simulink model "SkywalkerX8_Control_Observable_Feedback"  (R2018a)
settings: Solver=FixedStepAuto  StartTime=0.0  StopTime=120  FixedStep=0.001  RelTol=1e-3
undefined symbols (not defined in the file): DiscIntNeverNeededParam, magnitude, sigbuilder_block, SkywalkerX8
libraries: simulink_extras x13, sensors x7, simulink x5, sharedTrackingLibrary x2, dspmtrx3 x1
(part 1 of 3)
settings Model: Creator=David  LastModifiedBy=David
settings SolverCC: AlgebraicLoopSolver=LineSearch

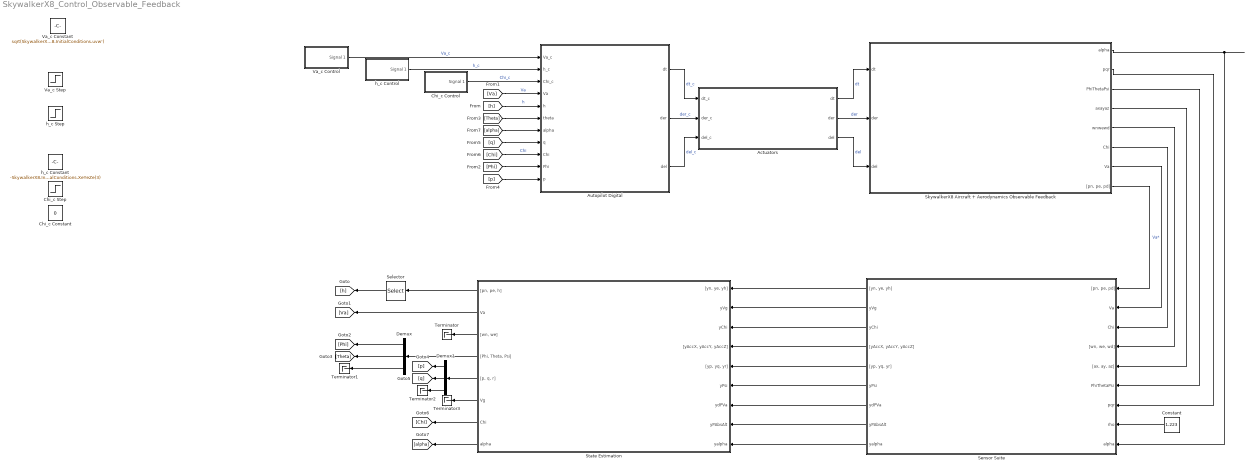
== system SkywalkerX8_Control_Observable_Feedback ==
  Actuators : Subsystem
      mask Display:
      | image('actuators.jpg', 'center')
      | 
      | color('white')
      | 
      | port_label('input', 1, 'd_{t_c} (Unitless)', 'texmode', 'on')
      | port_label('input', 2, 'd_{{er}_c} (rad)', 'texmode', 'on')
      | port_label('input', 3, 'd_{{el}_c} (rad)', 'texmode', 'on')
      | 
      | port_label('output', 1, 'd_t (Unitless)', 'texmode', 'on')
      | port_label('output', 2, 'd_{er} (rad)', 'texmode', 'on')
      | port_label('output', 3, 'd_{el} (rad)', 'texmode', 'on')
  Autopilot Digital : Subsystem
      mask Display:
      | image('autopilot.png', 'center')
      | 
      | port_label('output', 1, '\delta_t (Unitless)', 'texmode', 'on')
      | port_label('output', 2, '\delta_e_r (rad)', 'texmode', 'on')
      | port_label('output', 3, '\delta_e_l (rad)', 'texmode', 'on')
      | 
      | port_label('input', 1, 'V_{a_c} (m/s)', 'texmode', 'on')
      | port_label('input', 2, 'h_c (m)', 'texmode', 'on')
      | port_label('input', 3, '\chi_c (rad)', 'texmode', 'on')
      | port_label('input', 4, 'V_a (m/s)', 'texmode', 'on')
      | port_label('input', 5, 'Altitude (m)', 'texmode', 'on')
      | port_label('input', 6, '\theta (rad)', 'texmode', 'on')
      | port_label('input', 7, '\alpha (rad)', 'texmode', 'on')
      | port_label('input', 8, 'q (rad/s)', 'texmode', 'on')
      | port_label('input', 9, '\chi (rad)', 'texmode', 'on')
      | port_label('input', 10, '\phi (rad)', 'texmode', 'on')
      | port_label('input', 11, 'p (rad/s)', 'texmode', 'on')
  Chi_c Constant : Constant  Value=0
  Chi_c Control : Subsystem  Tag=STV Subsys  LoadFcn=sigbuilder_block('load');  StartFcn=sigbuilder_block('start');  StopFcn=sigbuilder_block('stop');  ClipboardFcn=sigbuilder_block('clipboard');  mask(Sigbuilder block){tuvar=[0:10]}
      mask help: Simulink:masks:SigbuilderBlock_MD
      mask init:
      | if ~strcmp(get_param(bdroot(gcbh),'SimulationStatus'),'stopped') tuvar = sigbuilder_block('maskInit'); end
      settings: CopyFcn=sigbuilder_block('copy');  DeleteFcn=sigbuilder_block('delete');  ModelCloseFcn=sigbuilder_block('modelClose');  PreSaveFcn=sigbuilder_block('preSave');  PauseFcn=sigbuilder_block('pause');  ContinueFcn=sigbuilder_block('continue');  NameChangeFcn=sigbuilder_block('namechange');  OpenFcn=sigbuilder_block('open',[437.6 199.2 550.4 400 ]);  CloseFcn=sigbuilder_block('close');
      mask Display: plot(0, 0, 100, 100,[2, 2, 32, 32, 2], [68, 8, 8, 68, 68],[32, 2], [38, 38], [32, 19, 2],[53, 60, 44], [32, 17, 17, 2],[16, 16, 31, 31]);txt = getActiveGroup(gcbh);text(2, 100, txt,'verticalAlignment', 'top');
  Chi_c Step : Step  After=deg2rad(90)  SampleTime=0
  Constant : Constant  Value=1.223
  Demux : Demux  Outputs=3
  Demux1 : Demux  Outputs=3
  Selector : Selector  InputPortWidth=3  IndexOptions=Index vector (dialog)  Indices=3  OutputSizes=1
  Sensor Suite : Subsystem
      mask Display:
      | image('telemetry.jpg')
      | 
      | color('cyan')
      | 
      | port_label('input', 1, '[p_N, p_E, p_D] (m)', 'texMode', 'On')
      | port_label('input', 2, 'V_a (m/s)', 'texMode', 'On')
      | port_label('input', 3, '\chi (rad)', 'texMode', 'On')
      | port_label('input', 4, '[w_N, w_E, w_D] (m/s)', 'texMode', 'On')
      | port_label('input', 5, '{\bfa_{inertial}} (m/s^2)', 'texMode', 'on')
      | port_label('input', 6, '[\phi, \theta, \psi] (rad)', 'texMode', 'on')
      | port_label('input', 7, '{\bf\omega_b} (rad/s)', 'texMode', 'on')
      | port_label('input', 8, '\rho (kg/m^3)', 'texMode', 'on')
      | port_label('input', 9, '\alpha (rad)', 'texMode', 'on')
      | 
      | port_label('output', 1, '[y_{GPS_N}, y_{GPS_E}, y_{GPS_h}] (m)', 'texMode', 'On')
      | port_label('output', 2, 'y_{GPS_{Vg}} (m/s)', 'texMode', 'On')
      | port_label('output', 3, 'y_{GPS_{\chi}} (rad)', 'texMode', 'On')
      | port_label('output', 4, '[y_{accel_x}, y_{accel_y}, y_{accel_z}] (m/s^2)', 'texMode', 'on')
      | port_label('output', 5, '[y_p, y_q, y_r] (rad/s)', 'texMode', 'on')
      | port_label('output', 6, 'y_{\psi} (rad)', 'texMode', 'on')
      | port_label('output', 7, 'y_{\DeltaP_{V_a}} (Pa)', 'texMode', 'on')
      | port_label('output', 8, 'y_{P_{abs}} (Pa)', 'texMode', 'on')
      | port_label('output', 9, 'y_\alpha (rad)', 'texMode', 'on')
  SkywalkerX8 Aircraft + Aerodynamics Observable Feedback : Subsystem
      mask Display:
      | image('x8SkySunset.png', 'center')
      | 
      | port_label('input', 1, '\delta_t (Unitless)', 'texmode', 'on')
      | port_label('input', 2, '\delta_e_r (rad)', 'texmode', 'on')
      | port_label('input', 3, '\delta_e_l (rad)', 'texmode', 'on')
      | 
      | port_label('output', 8, '[p_N, p_E, p_D] (m)', 'texMode', 'On')
      | port_label('output', 7, 'V_a (m/s)', 'texMode', 'On')
      | port_label('output', 6, '\chi (rad)', 'texMode', 'on')
      | port_label('output', 5, '[w_N, w_E, w_D] (m/s)', 'texMode', 'On')
      | port_label('output', 4, '{\bfa_{inertial}} (m/s^2)', 'texMode', 'on')
      | port_label('output', 3, '[\phi, \theta, \psi] (rad)', 'texMode', 'on')
      | port_label('output', 2, '{\bf\omega_b} (rad/s)', 'texMode', 'on')
      | port_label('output', 1, '\alpha (rad)', 'texMode', 'on')
  State Estimation : Subsystem
      mask Display:
      | image('state_estimate.jpg', 'center')
      | 
      | port_label('input', 1, '[y_{GPS_N}, y_{GPS_E}, y_{GPS_h}] (m)', 'texMode', 'On')
      | port_label('input', 2, 'y_{GPS_{Vg}} (m/s)', 'texMode', 'On')
      | port_label('input', 3, 'y_{GPS_{\chi}} (rad)', 'texMode', 'On')
      | port_label('input', 4, '[y_{accel_x}, y_{accel_y}, y_{accel_z}] (m/s^2)', 'texMode', 'on')
      | port_label('input', 5, '[y_p, y_q, y_r] (rad/s)', 'texMode', 'on')
      | port_label('input', 6, 'y_{\psi} (rad)', 'texMode', 'on')
      | port_label('input', 7, 'y_{\DeltaP_{V_a}} (Pa)', 'texMode', 'on')
      | port_label('input', 8, 'y_{P_{abs}} (Pa)', 'texMode', 'on')
      | port_label('input', 9, 'y_{\alpha} (rad)', 'texMode', 'on')
      | 
      | port_label('output', 1, '[p_N, p_E, h] (m)', 'texMode', 'On')
      | port_label('output', 2, 'V_a (m/s)', 'texMode', 'On')
      | port_label('output', 3, '[w_N, w_E] (m/s)', 'texMode', 'On')
      | port_label('output', 4, '[\phi, \theta, \psi] (rad)', 'texMode', 'on')
      | port_label('output', 5, '{\bf\omega_b} (rad/s)', 'texMode', 'on')
      | port_label('output', 6, 'V_g (m/s)', 'texMode', 'on')
      | port_label('output', 7, '\chi (rad)', 'texMode', 'on')
      | port_label('output', 8, '\alpha (rad)', 'texMode', 'on')
  Terminator{,1..3} (4 alike) : Terminator
  Va_c Constant : Constant  Value=sqrt(SkywalkerX8.InitialConditions.uvw*SkywalkerX8.InitialConditions.uvw')
  Va_c Control : Subsystem  Tag=STV Subsys  LoadFcn=sigbuilder_block('load');  StartFcn=sigbuilder_block('start');  StopFcn=sigbuilder_block('stop');  ClipboardFcn=sigbuilder_block('clipboard');  mask(Sigbuilder block){tuvar=[0:10]}
      mask help: Simulink:masks:SigbuilderBlock_MD
      mask init:
      | if ~strcmp(get_param(bdroot(gcbh),'SimulationStatus'),'stopped') tuvar = sigbuilder_block('maskInit'); end
      settings: CopyFcn=sigbuilder_block('copy');  DeleteFcn=sigbuilder_block('delete');  ModelCloseFcn=sigbuilder_block('modelClose');  PreSaveFcn=sigbuilder_block('preSave');  PauseFcn=sigbuilder_block('pause');  ContinueFcn=sigbuilder_block('continue');  NameChangeFcn=sigbuilder_block('namechange');  OpenFcn=sigbuilder_block('open',[437.6 199.2 550.4 400 ]);  CloseFcn=sigbuilder_block('close');
      mask Display: plot(0, 0, 100, 100,[2, 2, 32, 32, 2], [68, 8, 8, 68, 68],[32, 2], [38, 38], [32, 19, 2],[53, 60, 44], [32, 17, 17, 2],[16, 16, 31, 31]);txt = getActiveGroup(gcbh);text(2, 100, txt,'verticalAlignment', 'top');
  Va_c Step : Step  Before=sqrt(SkywalkerX8.InitialConditions.uvw*SkywalkerX8.InitialConditions.uvw')  After=sqrt(SkywalkerX8.InitialConditions.uvw*SkywalkerX8.InitialConditions.uvw')  SampleTime=0
  h_c Constant : Constant  Value=-SkywalkerX8.InitialConditions.XeYeZe(3)
  h_c Control : Subsystem  Tag=STV Subsys  LoadFcn=sigbuilder_block('load');  StartFcn=sigbuilder_block('start');  StopFcn=sigbuilder_block('stop');  ClipboardFcn=sigbuilder_block('clipboard');  mask(Sigbuilder block){tuvar=[0:10]}
      mask help: Simulink:masks:SigbuilderBlock_MD
      mask init:
      | if ~strcmp(get_param(bdroot(gcbh),'SimulationStatus'),'stopped') tuvar = sigbuilder_block('maskInit'); end
      settings: CopyFcn=sigbuilder_block('copy');  DeleteFcn=sigbuilder_block('delete');  ModelCloseFcn=sigbuilder_block('modelClose');  PreSaveFcn=sigbuilder_block('preSave');  PauseFcn=sigbuilder_block('pause');  ContinueFcn=sigbuilder_block('continue');  NameChangeFcn=sigbuilder_block('namechange');  OpenFcn=sigbuilder_block('open',[6 30 1428 771.75 ]);  CloseFcn=sigbuilder_block('close');
      mask Display: plot(0, 0, 100, 100,[2, 2, 32, 32, 2], [68, 8, 8, 68, 68],[32, 2], [38, 38], [32, 19, 2],[53, 60, 44], [32, 17, 17, 2],[16, 16, 31, 31]);txt = getActiveGroup(gcbh);text(2, 100, txt,'verticalAlignment', 'top');
  h_c Step : Step  Time=0.1  Before=-SkywalkerX8.InitialConditions.XeYeZe(3)  After=-2*SkywalkerX8.InitialConditions.XeYeZe(3)  SampleTime=0
  wires:
  Autopilot Digital/3(del) -> Actuators/3(del_c)  "del_c"
  Actuators/3(del) -> SkywalkerX8 Aircraft + Aerodynamics Observable Feedback/3(del)  "del"
  Actuators/2(der) -> SkywalkerX8 Aircraft + Aerodynamics Observable Feedback/2(der)  "der"
  Autopilot Digital/1(dt) -> Actuators/1(dt_c)  "dt_c"
  Chi_c Control/1(Signal 1) -> Autopilot Digital/3(Chi_c)  "Chi_c"
  Autopilot Digital/2(der) -> Actuators/2(der_c)  "der_c"
  h_c Control/1(Signal 1) -> Autopilot Digital/2(h_c)  "h_c"
  Actuators/1(dt) -> SkywalkerX8 Aircraft + Aerodynamics Observable Feedback/1(dt)  "dt"
  Va_c Control/1(Signal 1) -> Autopilot Digital/1(Va_c)  "Va_c"
  Sensor Suite/1("[yn, ye, yh]") -> State Estimation/1("[yn, ye, yh]")
  Sensor Suite/2(yVg) -> State Estimation/2(yVg)
  Sensor Suite/3(yChi) -> State Estimation/3(yChi)
  Sensor Suite/4("[yAccX, yAccY, yAccZ]") -> State Estimation/4("[yAccX, yAccY, yAccZ]")
  Sensor Suite/5("[yp, yq, yr]") -> State Estimation/5("[yp, yq, yr]")
  Sensor Suite/6(yPsi) -> State Estimation/6(yPsi)
  Sensor Suite/7(ydPVa) -> State Estimation/7(ydPVa)
  Sensor Suite/8(yPAbsAlt) -> State Estimation/8(yPAbsAlt)
  Sensor Suite/9(yalpha) -> State Estimation/9(yalpha)
  SkywalkerX8 Aircraft + Aerodynamics Observable Feedback/8("[pn, pe, pd]") -> Sensor Suite/1("[pn, pe, pd]")
  SkywalkerX8 Aircraft + Aerodynamics Observable Feedback/7(Va) -> Sensor Suite/2(Va)  "Va*"
  SkywalkerX8 Aircraft + Aerodynamics Observable Feedback/5(wnwewd) -> Sensor Suite/4("[wn, we, wd]")
  SkywalkerX8 Aircraft + Aerodynamics Observable Feedback/4(axayaz) -> Sensor Suite/5("[ax, ay, az]")
  SkywalkerX8 Aircraft + Aerodynamics Observable Feedback/3(PhiThetaPsi) -> Sensor Suite/6(PhiThetaPsi)
  SkywalkerX8 Aircraft + Aerodynamics Observable Feedback/2(pqr) -> Sensor Suite/7(pqr)
  SkywalkerX8 Aircraft + Aerodynamics Observable Feedback/1(alpha) -> Sensor Suite/9(alpha)
  Constant/1 -> Sensor Suite/8(rho)
  State Estimation/1("[pn, pe, h]") -> Selector/1
  Selector/1 -> [h]
  State Estimation/2(Va) -> [Va]
  State Estimation/3("[wn, we]") -> Terminator/1
  State Estimation/4("[Phi, Theta, Psi]") -> Demux/1
  Demux/1 -> [Phi]
  Demux/2 -> [Theta]
  Demux/3 -> Terminator1/1
  State Estimation/5("[p, q, r]") -> Demux1/1
  Demux1/1 -> [p]
  Demux1/2 -> [q]
  Demux1/3 -> Terminator2/1
  State Estimation/6(Vg) -> Terminator3/1
  State Estimation/7(Chi) -> [Chi]
  State Estimation/8(alpha) -> [alpha]
  [h] -> Autopilot Digital/5(h)  "h"
  [Va] -> Autopilot Digital/4(Va)  "Va"
  [Phi] -> Autopilot Digital/10(Phi)
  [Theta] -> Autopilot Digital/6(theta)
  [p] -> Autopilot Digital/11(p)
  [q] -> Autopilot Digital/8(q)
  [Chi] -> Autopilot Digital/9(Chi)  "Chi"
  [alpha] -> Autopilot Digital/7(alpha)
  SkywalkerX8 Aircraft + Aerodynamics Observable Feedback/6(Chi) -> Sensor Suite/3(Chi)

== system SkywalkerX8_Control_Observable_Feedback/Actuators ==
  dt_c : Inport
  der_c : Inport  Port=2
  del_c : Inport  Port=3
  Left Servo-Motor : Subsystem
      mask Display: image('servo.jpg', 'center')
  Motor Model : simulink_extras/Additional Linear/State-Space (with initial outputs)  A=SkywalkerX8.Actuators.Motor.SS.A  B=SkywalkerX8.Actuators.Motor.SS.B  C=SkywalkerX8.Actuators.Motor.SS.C  D=SkywalkerX8.Actuators.Motor.SS.D  U0=SkywalkerX8.InitialConditions.dt  Y0=SkywalkerX8.InitialConditions.dt  mask(State-Space with Initial Outputs){}
      settings: SourceProductName=Simulink  SourceProductBaseCode=SL
      mask Display: image('motor.jpg', 'center')
  Right Servo-Motor : Subsystem
      mask Display: image('servo.jpg', 'center')
  dt : Outport
  der : Outport  Port=2
  del : Outport  Port=3
  wires:
  del_c/1 -> Left Servo-Motor/1(del_c)
  Motor Model/1 -> dt/1
  Left Servo-Motor/1(del) -> del/1
  der_c/1 -> Right Servo-Motor/1(der_c)
  dt_c/1 -> Motor Model/1
  Right Servo-Motor/1(der) -> der/1

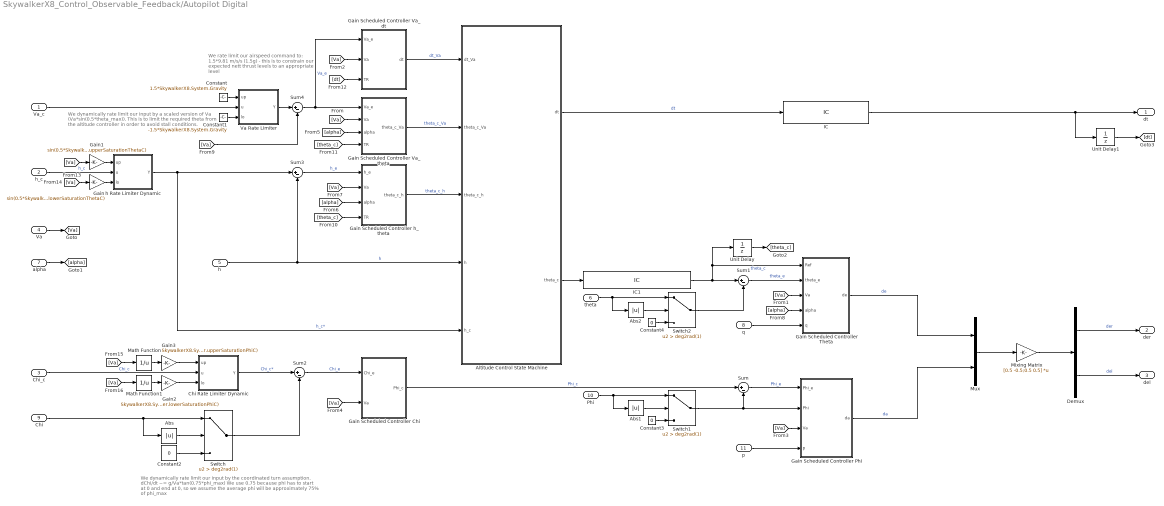
== system SkywalkerX8_Control_Observable_Feedback/Autopilot Digital ==
  note: We dynamically rate limit our input
      | by a scaled version of Va (Va*sin(0.5*theta_max)).
      |
      | This is to limit the required theta from the altitude controller
      | in order to avoid stall conditions.
  note: We dynamically rate limit our input
      | by the coordinated turn assumption.
      |
      | dChi/dt ~= g/Va*tan(0.75*phi_max)
      |
      | We use 0.75 because phi has to start at 0 and end at 0, so we assume
      | the average phi will be approximately 75% of phi_max
  note: We rate limit our airspeed command to:
      |
      | 1.5*9.81 m/s/s (1.5g) - this is to constrain our expected nett thrust levels to an appropriate level
  Va_c : Inport
  h_c : Inport  Port=2
  Chi_c : Inport  Port=3
  Va : Inport  Port=4
  h : Inport  Port=5
  theta : Inport  Port=6
  alpha : Inport  Port=7
  q : Inport  Port=8
  Chi : Inport  Port=9
  Phi : Inport  Port=10
  p : Inport  Port=11
  Abs : Abs
  Abs1 : Abs
  Abs2 : Abs
  Altitude Control State Machine : Stateflow chart  TreatAsAtomicUnit=on  mask{h_hold=SkywalkerX8.Control.Longitudinal.AltStateMachine.hHold, h_takeoff=SkywalkerX8.Control.Longitudinal.AltStateMachine.hTakeOff, theta_c_takeoff=SkywalkerX8.Control.Longitudinal.AltStateMachine.thetaTakeOff, hyst_frac=SkywalkerX8.Control.Longitudinal.AltStateMachine.HysteresisFraction, PreFlightBypass=SkywalkerX8.Control.Longitudinal.AltStateMachine.PreFlightBypass}
      mask prompts: h_hold "Altitude hold zone (+- band around the commanded altitude where theta will control altitude) (m)"; h_takeoff "Takeoff altitude (altitude after which we move away from constant pitch angle command) (m)"; theta_c_takeoff "Takeoff pitch angle (constant pitch angle at which to climb at at takeoff) (rad)"; hyst_frac "Hysteresis Fraction (Unitless)"; PreFlightBypass "Preflight Bypass (Unitless)"
  Chi Rate Limiter Dynamic : Subsystem  mask{initOutput=SkywalkerX8.InitialConditions.PhiThetaPsi(3)}
      mask prompts: initOutput "Initial output of dynamic rate limiter"
      mask DialogControl DescGroupVar Prompt: Rate Limiter Dynamic
      mask DialogControl DescTextVar Prompt: Limit rising and falling rates of the signals at the second input by using the first input (upper limit) and the third input (lower limit).
      mask Display:
      | image('rateLimit.png')
      | 
      | port_label('input', 1, 'up')
      | port_label('input', 2, 'u')
      | port_label('input', 3, 'lo')
      | 
      | port_label('output', 1, 'Y')
  Constant : Constant  Value=1.5*SkywalkerX8.System.Gravity
  Constant1 : Constant  Value=-1.5*SkywalkerX8.System.Gravity
  Constant2 : Constant  Value=0
  Constant3 : Constant  Value=0
  Constant4 : Constant  Value=0
  Demux : Demux  Outputs=2
  Gain : Gain  Gain=sin(0.5*SkywalkerX8.Control.Longitudinal.altController.lowerSaturationThetaC)
  Gain Scheduled Controller Chi : Subsystem
  Gain Scheduled Controller Phi : Subsystem
  Gain Scheduled Controller Theta : Subsystem
  Gain Scheduled Controller Va_dt : Subsystem
  Gain Scheduled Controller Va_theta : Subsystem
  Gain Scheduled Controller h_theta : Subsystem
  Gain1 : Gain  Gain=sin(0.5*SkywalkerX8.Control.Longitudinal.altController.upperSaturationThetaC)
  Gain2 : Gain  Gain=SkywalkerX8.System.Gravity*tan(0.75*SkywalkerX8.Control.Lateral.ChiController.lowerSaturationPhiC)
  Gain3 : Gain  Gain=SkywalkerX8.System.Gravity*tan(0.75*SkywalkerX8.Control.Lateral.ChiController.upperSaturationPhiC)
  IC : InitialCondition  Value=SkywalkerX8.InitialConditions.dt
  IC1 : InitialCondition  Value=SkywalkerX8.InitialConditions.PhiThetaPsi(2)
  Math Function : Math  Operator=reciprocal  SaturateOnIntegerOverflow=on
  Math Function1 : Math  Operator=reciprocal  SaturateOnIntegerOverflow=on
  Mixing Matrix : Gain  Gain=[0.5 -0.5;0.5 0.5]  Multiplication=Matrix(K*u)
  Mux : Mux  Inputs=2
  Sum{,1..4} (5 alike) : Sum  Inputs=|+-
  Switch : Switch  Criteria=u2 > Threshold  Threshold=deg2rad(1)
  Switch1 : Switch  Criteria=u2 > Threshold  Threshold=deg2rad(1)
  Switch2 : Switch  Criteria=u2 > Threshold  Threshold=deg2rad(1)
  Unit Delay : UnitDelay  InitialCondition=SkywalkerX8.InitialConditions.PhiThetaPsi(2)  SampleTime=SkywalkerX8.Control.Longitudinal.thetaController.Digital.SampleTime
  Unit Delay1 : UnitDelay  InitialCondition=SkywalkerX8.InitialConditions.dt  SampleTime=SkywalkerX8.Control.Longitudinal.VaDtController.Digital.SampleTime
  Va Rate Limiter : Subsystem  mask{initOutput=sqrt(SkywalkerX8.InitialConditions.uvw*SkywalkerX8.InitialConditions.uvw')}
      mask prompts: initOutput "Initial output of dynamic rate limiter"
      mask DialogControl DescGroupVar Prompt: Rate Limiter Dynamic
      mask DialogControl DescTextVar Prompt: Limit rising and falling rates of the signals at the second input by using the first input (upper limit) and the third input (lower limit).
      mask Display:
      | image('rateLimit.png')
      | 
      | port_label('input', 1, 'up')
      | port_label('input', 2, 'u')
      | port_label('input', 3, 'lo')
      | 
      | port_label('output', 1, 'Y')
  h Rate Limiter Dynamic : Subsystem  mask{initOutput=-SkywalkerX8.InitialConditions.XeYeZe(3)}
      mask prompts: initOutput "Initial output of dynamic rate limiter"
      mask DialogControl DescGroupVar Prompt: Rate Limiter Dynamic
      mask DialogControl DescTextVar Prompt: Limit rising and falling rates of the signals at the second input by using the first input (upper limit) and the third input (lower limit).
      mask Display:
      | image('rateLimit.png')
      | 
      | port_label('input', 1, 'up')
      | port_label('input', 2, 'u')
      | port_label('input', 3, 'lo')
      | 
      | port_label('output', 1, 'Y')
  dt : Outport
  der : Outport  Port=2
  del : Outport  Port=3
  wires:
  [Va] -> Sum4/2
  Sum4/1 -> Gain Scheduled Controller Va_theta/1(Va_e), Gain Scheduled Controller Va_dt/1(Va_e)  "Va_e"
  Demux/1 -> der/1  "der"
  Gain Scheduled Controller Chi/1(Phi_c) -> Sum/1  "Phi_c"
  h/1 -> Altitude Control State Machine/4(h), Sum3/2  "h"
  h Rate Limiter Dynamic/1(Y) -> Altitude Control State Machine/5(h_c), Sum3/1  "h_c*"
  Sum3/1 -> Gain Scheduled Controller h_theta/1(h_e)  "h_e"
  Sum2/1 -> Gain Scheduled Controller Chi/1(Chi_e)  "Chi_e"
  Switch1/1 -> Sum/2, Gain Scheduled Controller Phi/2(Phi)
  Sum/1 -> Gain Scheduled Controller Phi/1(Phi_e)  "Phi_e"
  Gain Scheduled Controller Phi/1(da) -> Mux/2  "da"
  [Va] -> Gain Scheduled Controller Phi/3(Va)
  [Va] -> Gain Scheduled Controller Theta/3(Va)
  Va_c/1 -> Va Rate Limiter/2(u)
  [alpha] -> Gain Scheduled Controller Va_theta/3(alpha)
  [Va] -> Gain Scheduled Controller Chi/2(Va)
  Sum1/1 -> Gain Scheduled Controller Theta/2(theta_e)  "theta_e"
  [Va] -> Gain Scheduled Controller Va_dt/2(Va)
  Demux/2 -> del/1  "del"
  alpha/1 -> [alpha]
  [Va] -> Gain Scheduled Controller Va_theta/2(Va)
  Chi/1 -> Abs/1, Switch/1
  Gain Scheduled Controller Theta/1(de) -> Mux/1  "de"
  p/1 -> Gain Scheduled Controller Phi/4(p)
  Va/1 -> [Va]
  Mux/1 -> Mixing Matrix/1
  Mixing Matrix/1 -> Demux/1
  [Va] -> Gain Scheduled Controller h_theta/2(Va)
  [alpha] -> Gain Scheduled Controller h_theta/3(alpha)
  Altitude Control State Machine/1(dt) -> IC/1  "dt"
  Gain Scheduled Controller Va_theta/1(theta_c_Va) -> Altitude Control State Machine/2(theta_c_Va)  "theta_c_Va"
  [theta_c] -> Gain Scheduled Controller Va_theta/4(TR)
  [dt] -> Gain Scheduled Controller Va_dt/3(TR)
  IC/1 -> Unit Delay1/1, dt/1
  [theta_c] -> Gain Scheduled Controller h_theta/4(TR)
  IC1/1 -> Unit Delay/1, Gain Scheduled Controller Theta/1(Ref), Sum1/1  "theta_c"
  [alpha] -> Gain Scheduled Controller Theta/4(alpha)
  q/1 -> Gain Scheduled Controller Theta/5(q)
  Gain Scheduled Controller h_theta/1(theta_c_h) -> Altitude Control State Machine/3(theta_c_h)  "theta_c_h"
  Altitude Control State Machine/2(theta_c) -> IC1/1
  Gain Scheduled Controller Va_dt/1(dt) -> Altitude Control State Machine/1(dt_Va)  "dt_Va"
  h_c/1 -> h Rate Limiter Dynamic/2(u)  "h_c"
  [Va] -> Gain1/1
  Gain/1 -> h Rate Limiter Dynamic/3(lo)
  [Va] -> Gain/1
  Gain1/1 -> h Rate Limiter Dynamic/1(up)
  [Va] -> Math Function1/1
  [Va] -> Math Function/1
  Gain2/1 -> Chi Rate Limiter Dynamic/3(lo)
  Gain3/1 -> Chi Rate Limiter Dynamic/1(up)
  Math Function/1 -> Gain3/1
  Math Function1/1 -> Gain2/1
  Va Rate Limiter/1(Y) -> Sum4/1
  Constant/1 -> Va Rate Limiter/1(up)
  Constant1/1 -> Va Rate Limiter/3(lo)
  Unit Delay/1 -> [theta_c]
  Unit Delay1/1 -> [dt]
  Abs/1 -> Switch/2
  Constant2/1 -> Switch/3
  Switch/1 -> Sum2/2
  Constant3/1 -> Switch1/3
  Abs1/1 -> Switch1/2
  Phi/1 -> Abs1/1, Switch1/1
  Constant4/1 -> Switch2/3
  Abs2/1 -> Switch2/2
  theta/1 -> Abs2/1, Switch2/1
  Switch2/1 -> Sum1/2
  Chi_c/1 -> Chi Rate Limiter Dynamic/2(u)  "Chi_c"
  Chi Rate Limiter Dynamic/1(Y) -> Sum2/1  "Chi_c*"

== system SkywalkerX8_Control_Observable_Feedback/Chi_c Control ==
  Demux : Demux  Tag=STV Demux  Outputs=1
  FromWs : FromWorkspace  Tag=STV FromWs  VariableName=tuvar  SampleTime=0
      SigBuilderData=|
      | common.afterFinalStr = 'Extrapolate'
      | common.sampleTime = 0
      | dataSet.timeRange = [0 120]
      | dataSet.name = 'Group 1'
      | sbobj.Groups.Name = 'Group 1'
      | sbobj.Groups.Signals.Name = 'Signal 1'
      | sbobj.Groups.Signals.XData = [0 10 10 35 35 55 55 90 90 120]
      | sbobj.Groups.Signals.YData = [0 0 1.5708 1.5708 0 0 1.5708 1.5708 0 0]
      | sbobj.Groups.TimeRange = [0 120]
  Signal 1 : Outport  Tag=STV Outport
  wires:
  Demux/1 -> Signal 1/1
  FromWs/1 -> Demux/1

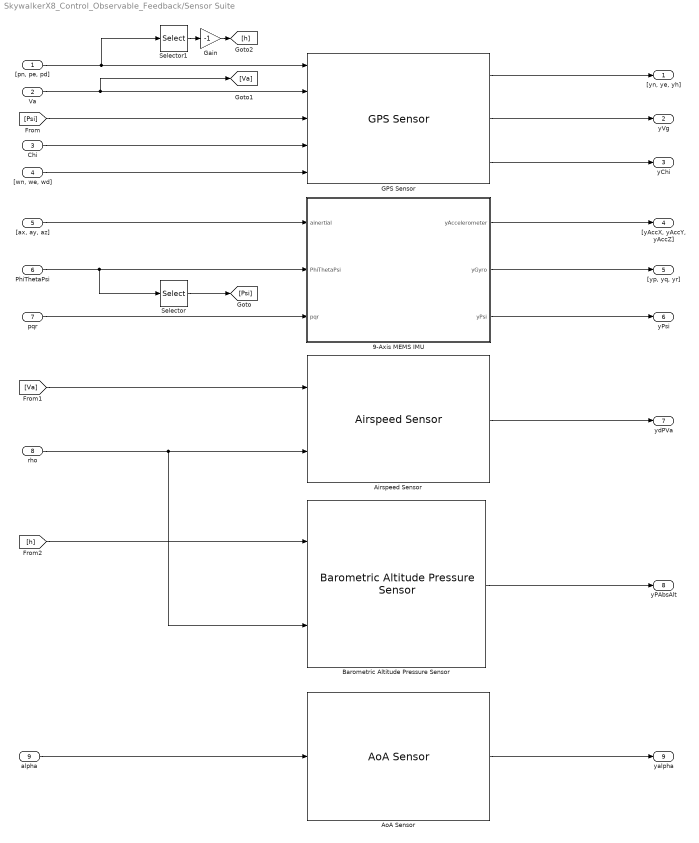
== system SkywalkerX8_Control_Observable_Feedback/Sensor Suite ==
  "[pn, pe, pd]" : Inport
  Va : Inport  Port=2
  Chi : Inport  Port=3
  "[wn, we, wd]" : Inport  Port=4
  "[ax, ay, az]" : Inport  Port=5
  PhiThetaPsi : Inport  Port=6
  pqr : Inport  Port=7
  rho : Inport  Port=8
  alpha : Inport  Port=9
  9-Axis MEMS IMU : Subsystem
      mask Display:
      | image('VNAV_IMU.jpg')
      | 
      | color('green')
      | 
      | port_label('input', 1, '{\bfa_{inertial}} (m/s^2)', 'texMode', 'on')
      | port_label('input', 2, '[\phi, \theta, \psi] (rad)', 'texMode', 'on')
      | port_label('input', 3, '{\bf\omega_b} (rad/s)', 'texMode', 'on')
      | 
      | port_label('output', 1, '[y_{accel_x}, y_{accel_y}, y_{accel_z}] (m/s^2)', 'texMode', 'on')
      | port_label('output', 2, '[y_p, y_q, y_r] (rad/s)', 'texMode', 'on')
      | port_label('output', 3, 'y_{\psi} (rad)', 'texMode', 'on')
  Airspeed Sensor : sensors/Airspeed Sensor  SampleTime=SkywalkerX8.Sensors.AirspeedPressure.SampleTime  diffPressureStdDev=SkywalkerX8.Sensors.AirspeedPressure.StdDev  diffPressureBandwidthHz=SkywalkerX8.Sensors.AirspeedPressure.BandwidthHz  diffPressureInit=SkywalkerX8.Sensors.AirspeedPressure.InitialCondition  diffPressureUpperSaturation=SkywalkerX8.Sensors.AirspeedPressure.UpperSat  diffPressureLowerSaturation=SkywalkerX8.Sensors.AirspeedPressure.LowerSat  diffPressureResolution=SkywalkerX8.Sensors.AirspeedPressure.Resolution
  AoA Sensor : sensors/AoA Sensor  SampleTime=SkywalkerX8.Sensors.AoA.SampleTime  alphaStdDev=SkywalkerX8.Sensors.AoA.StdDev  alphaBandwidthHz=SkywalkerX8.Sensors.AoA.BandwidthHz  alphaInit=SkywalkerX8.Sensors.AoA.InitialCondition  alphaUpperSaturation=SkywalkerX8.Sensors.AoA.UpperSat  alphaLowerSaturation=SkywalkerX8.Sensors.AoA.LowerSat  alphaResolution=SkywalkerX8.Sensors.AoA.Resolution
  Barometric Altitude Pressure Sensor : sensors/Barometric Altitude Pressure Sensor  g=SkywalkerX8.System.Gravity  SampleTime=SkywalkerX8.Sensors.AltitudePressure.SampleTime  absPressureStdDev=SkywalkerX8.Sensors.AltitudePressure.StdDev  absPressureBandwidthHz=SkywalkerX8.Sensors.AltitudePressure.BandwidthHz  absPressureInit=SkywalkerX8.Sensors.AltitudePressure.InitialCondition  absPressureUpperSaturation=SkywalkerX8.Sensors.AltitudePressure.UpperSat  absPressureLowerSaturation=SkywalkerX8.Sensors.AltitudePressure.LowerSat  absPressureResolution=SkywalkerX8.Sensors.AltitudePressure.Resolution
  GPS Sensor : sensors/GPS Sensor  SampleTime=SkywalkerX8.Sensors.GPS.SampleTime  pnInit=SkywalkerX8.Sensors.GPS.pnInit  peInit=SkywalkerX8.Sensors.GPS.peInit  pdInit=SkywalkerX8.Sensors.GPS.pdInit  VgInit=SkywalkerX8.Sensors.GPS.VgInit  ChiInit=SkywalkerX8.Sensors.GPS.ChiInit  GPSNStdDev=SkywalkerX8.Sensors.GPS.North.StdDev  OneOverkGPSN=SkywalkerX8.Sensors.GPS.North.TimeConstant  GPSEStdDev=SkywalkerX8.Sensors.GPS.East.StdDev  OneOverkGPSE=SkywalkerX8.Sensors.GPS.East.TimeConstant  GPSAltStdDev=SkywalkerX8.Sensors.GPS.Alt.StdDev  OneOverkGPSAlt=SkywalkerX8.Sensors.GPS.Alt.TimeConstant  GPSVStdDev=SkywalkerX8.Sensors.GPS.Velocity.StdDev
  Gain : Gain  Gain=-1
  Selector : Selector  InputPortWidth=3  IndexOptions=Index vector (dialog)  Indices=3  OutputSizes=1
  Selector1 : Selector  InputPortWidth=3  IndexOptions=Index vector (dialog)  Indices=3  OutputSizes=1
  "[yn, ye, yh]" : Outport
  yVg : Outport  Port=2
  yChi : Outport  Port=3
  "[yAccX, yAccY, yAccZ]" : Outport  Port=4
  "[yp, yq, yr]" : Outport  Port=5
  yPsi : Outport  Port=6
  ydPVa : Outport  Port=7
  yPAbsAlt : Outport  Port=8
  yalpha : Outport  Port=9
  wires:
  "[pn, pe, pd]"/1 -> GPS Sensor/1, Selector1/1
  Va/1 -> [Va], GPS Sensor/2
  PhiThetaPsi/1 -> 9-Axis MEMS IMU/2(PhiThetaPsi), Selector/1
  Airspeed Sensor/1 -> ydPVa/1
  [Psi] -> GPS Sensor/3
  Selector1/1 -> Gain/1
  rho/1 -> Barometric Altitude Pressure Sensor/2, Airspeed Sensor/2
  GPS Sensor/3 -> yChi/1
  Selector/1 -> [Psi]
  [h] -> Barometric Altitude Pressure Sensor/1
  9-Axis MEMS IMU/3(yPsi) -> yPsi/1
  [Va] -> Airspeed Sensor/1
  pqr/1 -> 9-Axis MEMS IMU/3(pqr)
  9-Axis MEMS IMU/2(yGyro) -> "[yp, yq, yr]"/1
  "[wn, we, wd]"/1 -> GPS Sensor/5
  Barometric Altitude Pressure Sensor/1 -> yPAbsAlt/1
  GPS Sensor/1 -> "[yn, ye, yh]"/1
  Gain/1 -> [h]
  GPS Sensor/2 -> yVg/1
  "[ax, ay, az]"/1 -> 9-Axis MEMS IMU/1(ainertial)
  9-Axis MEMS IMU/1(yAccelerometer) -> "[yAccX, yAccY, yAccZ]"/1
  AoA Sensor/1 -> yalpha/1
  alpha/1 -> AoA Sensor/1
  Chi/1 -> GPS Sensor/4

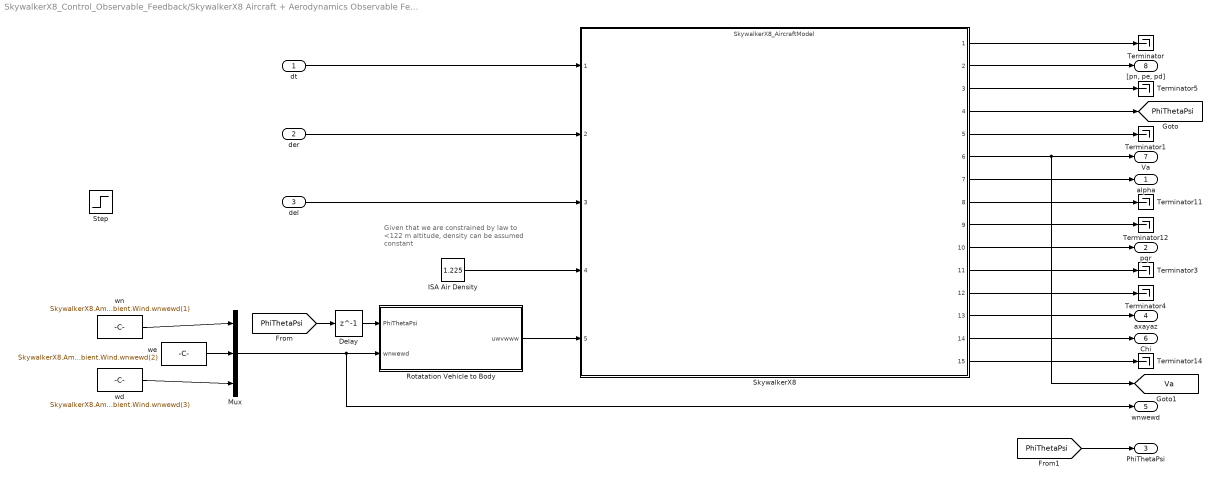
== system SkywalkerX8_Control_Observable_Feedback/SkywalkerX8 Aircraft + Aerodynamics Observable Feedback ==
  note: Given that we are constrained by law to
      | <122 m altitude, density can be assumed
      | constant
  dt : Inport
  der : Inport  Port=2
  del : Inport  Port=3
  Delay : Delay  DelayLength=1  InitialCondition=SkywalkerX8.InitialConditions.PhiThetaPsi
  ISA Air Density : Constant  Value=1.225
  Mux : Mux  Inputs=3
  Rotatation Vehicle to Body : MATLAB Function  TreatAsAtomicUnit=on
  SkywalkerX8 : ModelReference  ModelNameDialog=SkywalkerX8_AircraftModel  ModelReferenceVersion=1.361
      mask Display:
      | image('C:\MATLAB\masters\icons\Skywalker Main Block Icon.png', 'center')
      | 
      | color('cyan')
      | 
      | port_label('input', 1, 'k_{motor} (Unitless)', 'texmode', 'on')
      | port_label('input', 2, '\delta_{er} (rad)', 'texmode', 'on')
      | port_label('input', 3, '\delta_{el} (rad)', 'texmode', 'on')
      | port_label('input', 4, '\rho (kg/m^3)', 'texmode', 'on')
      | port_label('input', 5, '{\bf V_w^b} (m/s)', 'texmode', 'on')
      | 
      | port_label('output', 1, '{\bf V_e} (m/s)', 'texmode', 'on')
      | port_label('output', 2, '{\bf X_e} (m)', 'texmode', 'on')
      | port_label('output', 3, 'Altitude (m)', 'texmode', 'on')
      | port_label('output', 4, '\phi \theta \psi (rad)', 'texmode', 'on')
      | port_label('output', 5, 'R_{inertial}^{body}', 'texmode', 'on')
      | port_label('output', 6, 'V_a (m/s)', 'texmode', 'on')
      | port_label('output', 7, 'alpha (rad)', 'texmode', 'on')
      | port_label('output', 8, 'beta (rad)', 'texmode', 'on')
      | port_label('output', 9, '{\bf V_b} (m/s)', 'texmode', 'on')
      | port_label('output', 10, '{\bf \omega_b} (rad/s)', 'texmode', 'on')
      | port_label('output', 11, '{\bf \delta\omega_b/\deltat} (rad/s^2)', 'texmode', 'on')
      | port_label('output', 12, '{\bf a_{body}} (m/s^2)', 'texmode', 'on')
      | port_label('output', 13, '{\bf a_{inertial}} (m/s^2)', 'texmode', 'on')
      | port_label('output', 14, '\chi (rad)', 'texmode', 'on')
      | port_label('output', 15, '\chi_c (rad)', 'texmode', 'on')
  Step : Step  Time=30  Before=SkywalkerX8.Ambient.Wind.wnwewd(2)  After=9  SampleTime=0
  Terminator{,1,3..5,11..12,14} (8 alike) : Terminator
  wd : Constant  Value=SkywalkerX8.Ambient.Wind.wnwewd(3)
  we : Constant  Value=SkywalkerX8.Ambient.Wind.wnwewd(2)
  wn : Constant  Value=SkywalkerX8.Ambient.Wind.wnwewd(1)
  alpha : Outport
  pqr : Outport  Port=2
  PhiThetaPsi : Outport  Port=3
  axayaz : Outport  Port=4
  wnwewd : Outport  Port=5
  Chi : Outport  Port=6
  Va : Outport  Port=7
  "[pn, pe, pd]" : Outport  Port=8
  tag scope: PhiThetaPsi=global, Va=global
  wires:
  SkywalkerX8/12 -> Terminator4/1
  SkywalkerX8/13 -> axayaz/1
  Rotatation Vehicle to Body/1(uwvwww) -> SkywalkerX8/5
  SkywalkerX8/11 -> Terminator3/1
  SkywalkerX8/6 -> [Va], Va/1
  SkywalkerX8/1 -> Terminator/1
  SkywalkerX8/5 -> Terminator1/1
  SkywalkerX8/7 -> alpha/1
  dt/1 -> SkywalkerX8/1
  SkywalkerX8/8 -> Terminator11/1
  SkywalkerX8/3 -> Terminator5/1
  SkywalkerX8/9 -> Terminator12/1
  SkywalkerX8/2 -> "[pn, pe, pd]"/1
  SkywalkerX8/4 -> [PhiThetaPsi]
  SkywalkerX8/15 -> Terminator14/1
  SkywalkerX8/10 -> pqr/1
  ISA Air Density/1 -> SkywalkerX8/4
  SkywalkerX8/14 -> Chi/1
  del/1 -> SkywalkerX8/3
  der/1 -> SkywalkerX8/2
  Mux/1 -> wnwewd/1, Rotatation Vehicle to Body/2(wnwewd)
  [PhiThetaPsi] -> Delay/1
  [PhiThetaPsi] -> PhiThetaPsi/1
  Delay/1 -> Rotatation Vehicle to Body/1(PhiThetaPsi)
  we/1 -> Mux/2
  wn/1 -> Mux/1
  wd/1 -> Mux/3

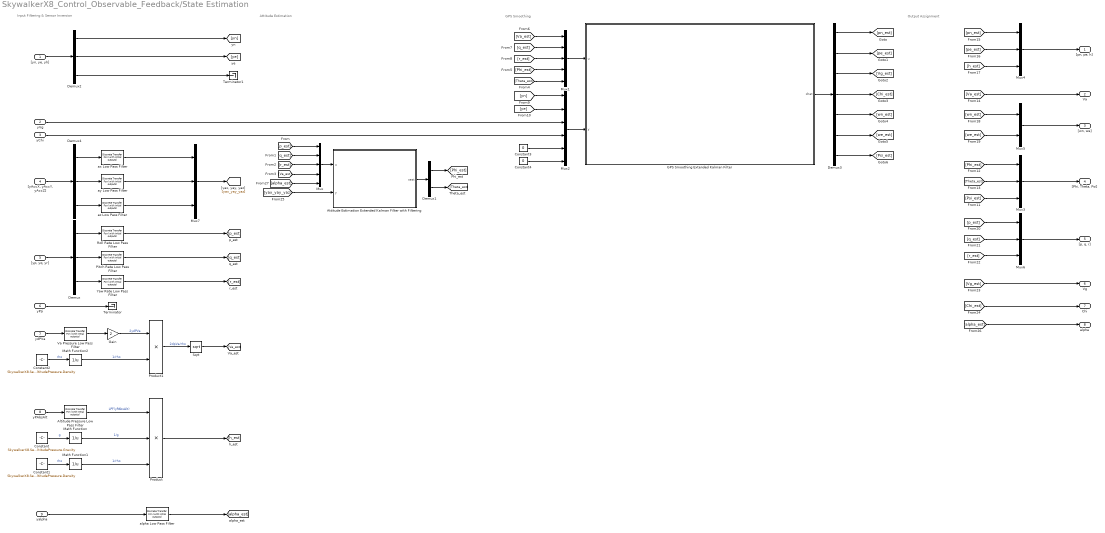
== system SkywalkerX8_Control_Observable_Feedback/State Estimation ==
  note: Output Assignment
  note: GPS Smoothing
  note: Attitude Estimation
  note: Input Filtering & Sensor Inversion
  "[yn, ye, yh]" : Inport  PortDimensions=3
  yVg : Inport  Port=2
  yChi : Inport  Port=3
  "[yAccX, yAccY, yAccZ]" : Inport  Port=4  PortDimensions=3
  "[yp, yq, yr]" : Inport  Port=5  PortDimensions=3
  yPsi : Inport  Port=6
  ydPVa : Inport  Port=7
  yPAbsAlt : Inport  Port=8
  yalpha : Inport  Port=9
  Altitude Pressure Low Pass Filter : simulink_extras/Additional Discrete/Discrete Transfer Fcn (with initial outputs)  N=cell2mat(SkywalkerX8.Sensors.Filters.AltitudePressure.FilterTFDigital.Numerator)  D=cell2mat(SkywalkerX8.Sensors.Filters.AltitudePressure.FilterTFDigital.Denominator)  U0=SkywalkerX8.Sensors.Filters.AltitudePressure.InitialCondition  Y0=SkywalkerX8.Sensors.Filters.AltitudePressure.InitialCondition  TS=SkywalkerX8.Sensors.Filters.AltitudePressure.FilterSampleTime
      settings: SourceProductName=Simulink  SourceProductBaseCode=SL
  Attitude Estimation Extended Kalman Filter with Filtering : Subsystem
      mask Display:
      | port_label('input', 1, '{\bf u} = [p, q, r, V_a, \alpha]', 'texMode', 'On')
      | port_label('input', 2, '{\bf y} = [a_x, a_y, a_z]', 'texMode', 'On')
      | 
      | port_label('output', 1, '{\bf x_{est}} = [\Phi, \theta]', 'texMode', 'On')
  Constant : Constant  Value=SkywalkerX8.Sensors.StateEstimate.SensorInversion.AltitudePressure.Gravity
  Constant1 : Constant  Value=SkywalkerX8.Sensors.StateEstimate.SensorInversion.AltitudePressure.Density
  Constant2 : Constant  Value=SkywalkerX8.Sensors.StateEstimate.SensorInversion.AltitudePressure.Density
  Constant3 : Constant  Value=0
  Constant4 : Constant  Value=0
  Demux : Demux  Outputs=3
  Demux1 : Demux  Outputs=2
  Demux2 : Demux  Outputs=3
  Demux3 : Demux  Outputs=7
  Demux4 : Demux  Outputs=3
  GPS Smoothing Extended Kalman Filter : Subsystem
      mask Display:
      | port_label('input', 1, '{\bf u} = [V_a, q, r, \Phi, \theta]', 'texMode', 'On')
      | port_label('input', 2, '{\bf y} = [y_{GPS_N}, y_{GPS_E}, y_{GPS_{V_g}}, y_{GPS_\chi}, y_{GPS_{wind_N}}, y_{GPS_{wind_E}}]', 'texMode', 'On')
      | 
      | port_label('output', 1, '{\bf x_{est}} = [p_n, p_e, V_g, \chi, w_n, w_e, \psi]', 'texMode', 'On')
  Gain : Gain  Gain=2
  Math Function : Math  Operator=reciprocal  SaturateOnIntegerOverflow=on
  Math Function1 : Math  Operator=reciprocal  SaturateOnIntegerOverflow=on
  Math Function2 : Math  Operator=reciprocal  SaturateOnIntegerOverflow=on
  Mux : Mux  Inputs=5
  Mux1 : Mux  Inputs=5
  Mux2 : Mux  Inputs=6
  Mux{3..4,6..7} (4 alike) : Mux  Inputs=3
  Mux5 : Mux  Inputs=2
  Pitch Rate Low Pass Filter : simulink_extras/Additional Discrete/Discrete Transfer Fcn (with initial outputs)  N=cell2mat(SkywalkerX8.Sensors.Filters.AngularRates.Pitch.FilterTFDigital.Numerator)  D=cell2mat(SkywalkerX8.Sensors.Filters.AngularRates.Pitch.FilterTFDigital.Denominator)  U0=SkywalkerX8.Sensors.Filters.AngularRates.Pitch.InitialCondition  Y0=SkywalkerX8.Sensors.Filters.AngularRates.Pitch.InitialCondition  TS=SkywalkerX8.Sensors.Filters.AngularRates.Pitch.FilterSampleTime
      settings: SourceProductName=Simulink  SourceProductBaseCode=SL
  Product : Product  Inputs=3
  Product1 : Product
  Roll Rate Low Pass Filter : simulink_extras/Additional Discrete/Discrete Transfer Fcn (with initial outputs)  N=cell2mat(SkywalkerX8.Sensors.Filters.AngularRates.Roll.FilterTFDigital.Numerator)  D=cell2mat(SkywalkerX8.Sensors.Filters.AngularRates.Roll.FilterTFDigital.Denominator)  U0=SkywalkerX8.Sensors.Filters.AngularRates.Roll.InitialCondition  Y0=SkywalkerX8.Sensors.Filters.AngularRates.Roll.InitialCondition  TS=SkywalkerX8.Sensors.Filters.AngularRates.Roll.FilterSampleTime
      settings: SourceProductName=Simulink  SourceProductBaseCode=SL
  Sqrt : Sqrt  SaturateOnIntegerOverflow=on
  Terminator : Terminator
  Terminator1 : Terminator
  Va Pressure Low Pass Filter : simulink_extras/Additional Discrete/Discrete Transfer Fcn (with initial outputs)  N=cell2mat(SkywalkerX8.Sensors.Filters.AirspeedPressure.FilterTFDigital.Numerator)  D=cell2mat(SkywalkerX8.Sensors.Filters.AirspeedPressure.FilterTFDigital.Denominator)  U0=SkywalkerX8.Sensors.Filters.AirspeedPressure.InitialCondition  Y0=SkywalkerX8.Sensors.Filters.AirspeedPressure.InitialCondition  TS=SkywalkerX8.Sensors.Filters.AirspeedPressure.FilterSampleTime
      settings: SourceProductName=Simulink  SourceProductBaseCode=SL
  Yaw Rate Low Pass Filter : simulink_extras/Additional Discrete/Discrete Transfer Fcn (with initial outputs)  N=cell2mat(SkywalkerX8.Sensors.Filters.AngularRates.Yaw.FilterTFDigital.Numerator)  D=cell2mat(SkywalkerX8.Sensors.Filters.AngularRates.Yaw.FilterTFDigital.Denominator)  U0=SkywalkerX8.Sensors.Filters.AngularRates.Yaw.InitialCondition  Y0=SkywalkerX8.Sensors.Filters.AngularRates.Yaw.InitialCondition  TS=SkywalkerX8.Sensors.Filters.AngularRates.Yaw.FilterSampleTime
      settings: SourceProductName=Simulink  SourceProductBaseCode=SL
  alpha Low Pass Filter : simulink_extras/Additional Discrete/Discrete Transfer Fcn (with initial outputs)  N=cell2mat(SkywalkerX8.Sensors.Filters.AoA.FilterTFDigital.Numerator)  D=cell2mat(SkywalkerX8.Sensors.Filters.AoA.FilterTFDigital.Denominator)  U0=SkywalkerX8.Sensors.Filters.AoA.InitialCondition  Y0=SkywalkerX8.Sensors.Filters.AoA.InitialCondition  TS=SkywalkerX8.Sensors.Filters.AoA.FilterSampleTime
      settings: SourceProductName=Simulink  SourceProductBaseCode=SL
  ax Low Pass Filter : simulink_extras/Additional Discrete/Discrete Transfer Fcn (with initial outputs)  N=cell2mat(SkywalkerX8.Sensors.EKF.Attitude.Filters.axFilterTFDigital.Numerator)  D=cell2mat(SkywalkerX8.Sensors.EKF.Attitude.Filters.axFilterTFDigital.Denominator)  U0=SkywalkerX8.Sensors.EKF.Attitude.InitialMeasurement(1)  Y0=SkywalkerX8.Sensors.EKF.Attitude.InitialMeasurement(1)  TS=SkywalkerX8.Sensors.EKF.Attitude.Filters.aFilterSampleTime
      settings: SourceProductName=Simulink  SourceProductBaseCode=SL
  ay Low Pass Filter : simulink_extras/Additional Discrete/Discrete Transfer Fcn (with initial outputs)  N=cell2mat(SkywalkerX8.Sensors.EKF.Attitude.Filters.ayFilterTFDigital.Numerator)  D=cell2mat(SkywalkerX8.Sensors.EKF.Attitude.Filters.ayFilterTFDigital.Denominator)  U0=SkywalkerX8.Sensors.EKF.Attitude.InitialMeasurement(2)  Y0=SkywalkerX8.Sensors.EKF.Attitude.InitialMeasurement(2)  TS=SkywalkerX8.Sensors.EKF.Attitude.Filters.aFilterSampleTime
      settings: SourceProductName=Simulink  SourceProductBaseCode=SL
  az Low Pass Filter : simulink_extras/Additional Discrete/Discrete Transfer Fcn (with initial outputs)  N=cell2mat(SkywalkerX8.Sensors.EKF.Attitude.Filters.azFilterTFDigital.Numerator)  D=cell2mat(SkywalkerX8.Sensors.EKF.Attitude.Filters.azFilterTFDigital.Denominator)  U0=SkywalkerX8.Sensors.EKF.Attitude.InitialMeasurement(3)  Y0=SkywalkerX8.Sensors.EKF.Attitude.InitialMeasurement(3)  TS=SkywalkerX8.Sensors.EKF.Attitude.Filters.aFilterSampleTime
      settings: SourceProductName=Simulink  SourceProductBaseCode=SL
  "[pn, pe, h]" : Outport
  Va : Outport  Port=2
  "[wn, we]" : Outport  Port=3
  "[Phi, Theta, Psi]" : Outport  Port=4
  "[p, q, r]" : Outport  Port=5
  Vg : Outport  Port=6
  Chi : Outport  Port=7
  alpha : Outport  Port=8
  wires:
  [Phi_est] -> Mux1/4
  Math Function1/1 -> Product/3  "1/rho"
  [ye] -> Mux2/2
  Sqrt/1 -> [Va_est]
  Demux/2 -> Pitch Rate Low Pass Filter/1
  [r_est] -> Mux/3
  Math Function2/1 -> Product1/2  "1/rho"
  yChi/1 -> Mux2/4
  Demux2/3 -> Terminator1/1
  Mux4/1 -> "[pn, pe, h]"/1
  Mux6/1 -> "[p, q, r]"/1
  [r_est] -> Mux1/3
  Constant3/1 -> Mux2/5
  Constant2/1 -> Math Function2/1  "rho"
  Demux3/4 -> [Chi_est]
  Demux3/3 -> [Vg_est]
  [h_est] -> Mux4/3
  Math Function/1 -> Product/2  "1/g"
  [we_est] -> Mux5/2
  "[yp, yq, yr]"/1 -> Demux/1
  [Theta_est] -> Mux1/5
  Demux3/7 -> [Psi_est]
  Mux2/1 -> GPS Smoothing Extended Kalman Filter/2(y)
  Constant4/1 -> Mux2/6
  [r_est] -> Mux6/3
  Mux/1 -> Attitude Estimation Extended Kalman Filter with Filtering/1(u)
  [wn_est] -> Mux5/1
  Demux2/2 -> [ye]
  GPS Smoothing Extended Kalman Filter/1(xhat) -> Demux3/1
  Constant1/1 -> Math Function1/1  "rho"
  Demux2/1 -> [yn]
  Demux3/6 -> [we_est]
  [q_est] -> Mux6/2
  "[yAccX, yAccY, yAccZ]"/1 -> Demux4/1
  Demux1/2 -> [Theta_est]
  Mux1/1 -> GPS Smoothing Extended Kalman Filter/1(u)
  Demux3/5 -> [wn_est]
  Attitude Estimation Extended Kalman Filter with Filtering/1(xest) -> Demux1/1
  Gain/1 -> Product1/1  "2ydPVa"
  Constant/1 -> Math Function/1  "g"
  [p_est] -> Mux/1
  yVg/1 -> Mux2/3
  Altitude Pressure Low Pass Filter/1 -> Product/1  "LPF(yPAbsAlt)"
  [Chi_est] -> Chi/1
  yPsi/1 -> Terminator/1
  [q_est] -> Mux1/2
  Demux3/1 -> [pn_est]
  [Va_est] -> Mux1/1
  [Theta_est] -> Mux3/2
  Va Pressure Low Pass Filter/1 -> Gain/1
  [q_est] -> Mux/2
  Product1/1 -> Sqrt/1  "2dpVa/rho"
  Yaw Rate Low Pass Filter/1 -> [r_est]
  Product/1 -> [h_est]
  [Va_est] -> Mux/4
  ydPVa/1 -> Va Pressure Low Pass Filter/1
  [Psi_est] -> Mux3/3
  Pitch Rate Low Pass Filter/1 -> [q_est]
  Demux/1 -> Roll Rate Low Pass Filter/1
  yPAbsAlt/1 -> Altitude Pressure Low Pass Filter/1
  Demux/3 -> Yaw Rate Low Pass Filter/1
  [pn_est] -> Mux4/1
  [p_est] -> Mux6/1
  Demux3/2 -> [pe_est]
  Demux1/1 -> [Phi_est]
  [Vg_est] -> Vg/1
  "[yn, ye, yh]"/1 -> Demux2/1
  [pe_est] -> Mux4/2
  [Phi_est] -> Mux3/1
  Mux3/1 -> "[Phi, Theta, Psi]"/1
  Mux5/1 -> "[wn, we]"/1
  [Va_est] -> Va/1
  [yn] -> Mux2/1
  Roll Rate Low Pass Filter/1 -> [p_est]
  Demux4/1 -> ax Low Pass Filter/1
  Demux4/2 -> ay Low Pass Filter/1
  Demux4/3 -> az Low Pass Filter/1
  ax Low Pass Filter/1 -> Mux7/1
  ay Low Pass Filter/1 -> Mux7/2
  az Low Pass Filter/1 -> Mux7/3
  Mux7/1 -> [yax_yay_yaz]
  [yax_yay_yaz] -> Attitude Estimation Extended Kalman Filter with Filtering/2(y)
  yalpha/1 -> alpha Low Pass Filter/1
  alpha Low Pass Filter/1 -> [alpha_est]
  [alpha_est] -> alpha/1
  [alpha_est] -> Mux/5

== system SkywalkerX8_Control_Observable_Feedback/Va_c Control ==
  Demux : Demux  Tag=STV Demux  Outputs=1
  FromWs : FromWorkspace  Tag=STV FromWs  VariableName=tuvar  SampleTime=0
      SigBuilderData=|
      | common.afterFinalStr = 'Extrapolate'
      | common.sampleTime = 0
      | dataSet.timeRange = [0 120]
      | dataSet.name = 'Group 1'
      | sbobj.Groups.Name = 'Group 1'
      | sbobj.Groups.Signals.Name = 'Signal 1'
      | sbobj.Groups.Signals.XData = [0 10 10 30 30 50 50 80 80 120]
      | sbobj.Groups.Signals.YData = [17.3072 17.3 20 20 17.3072 17.3072 15 15 17.3072 17.3072]
      | sbobj.Groups.TimeRange = [0 120]
  Signal 1 : Outport  Tag=STV Outport
  wires:
  Demux/1 -> Signal 1/1
  FromWs/1 -> Demux/1

== system SkywalkerX8_Control_Observable_Feedback/h_c Control ==
  Demux : Demux  Tag=STV Demux  Outputs=1
  FromWs : FromWorkspace  Tag=STV FromWs  VariableName=tuvar  SampleTime=0
      SigBuilderData=|
      | common.afterFinalStr = 'Extrapolate'
      | common.sampleTime = 0
      | dataSet.timeRange = [0 120]
      | dataSet.name = 'Group 1'
      | sbobj.Groups.Name = 'Group 1'
      | sbobj.Groups.Signals.Name = 'Signal 1'
      | sbobj.Groups.Signals.XData = [0 1 1 20 20 40 40 60 80 80 100 100 120]
      | sbobj.Groups.Signals.YData = [50 50 60 60 75 75 100 100 80 60 60 100 100]
      | sbobj.Groups.TimeRange = [0 120]
  Signal 1 : Outport  Tag=STV Outport
  wires:
  Demux/1 -> Signal 1/1
  FromWs/1 -> Demux/1

== system SkywalkerX8_Control_Observable_Feedback/Actuators/Left Servo-Motor ==
  del_c : Inport
  Abs : Abs
  Compare To Constant : simulink/Logic and Bit Operations/Compare To Constant  relop=>  const=SkywalkerX8.Actuators.Servos.RateLimit  OutDataTypeStr=boolean
  Derivative : Derivative
  Rate Limiter : RateLimiter  Commented=through  RisingSlewLimit=SkywalkerX8.Actuators.Servos.RateLimit  FallingSlewLimit=-SkywalkerX8.Actuators.Servos.RateLimit  SampleTimeMode=inherited  InitialCondition=SkywalkerX8.InitialConditions.de*0.5 + SkywalkerX8.InitialConditions.da*0.5
  Saturation : Saturate  UpperLimit=SkywalkerX8.Actuators.Servos.UpperSaturation  LowerLimit=SkywalkerX8.Actuators.Servos.LowerSaturation
  Second Order Servo-Motor Model : simulink_extras/Additional Linear/State-Space (with initial outputs)  A=SkywalkerX8.Actuators.Servos.SS.A  B=SkywalkerX8.Actuators.Servos.SS.B  C=SkywalkerX8.Actuators.Servos.SS.C  D=SkywalkerX8.Actuators.Servos.SS.D  U0=(SkywalkerX8.InitialConditions.de*0.5 + SkywalkerX8.InitialConditions.da*0.5)  Y0=(SkywalkerX8.InitialConditions.de*0.5 + SkywalkerX8.InitialConditions.da*0.5)
      settings: SourceProductName=Simulink  SourceProductBaseCode=SL
  Terminator : Terminator
  del : Outport
  wires:
  Rate Limiter/1 -> Saturation/1
  del_c/1 -> Second Order Servo-Motor Model/1
  Saturation/1 -> del/1
  Derivative/1 -> Abs/1
  Abs/1 -> Compare To Constant/1
  Compare To Constant/1 -> Terminator/1  "lServoRateLimitCheck"
  Second Order Servo-Motor Model/1 -> Derivative/1, Rate Limiter/1

== system SkywalkerX8_Control_Observable_Feedback/Actuators/Right Servo-Motor ==
  der_c : Inport
  Abs : Abs
  Compare To Constant : simulink/Logic and Bit Operations/Compare To Constant  relop=>  const=SkywalkerX8.Actuators.Servos.RateLimit  OutDataTypeStr=boolean
  Derivative : Derivative
  Rate Limiter : RateLimiter  Commented=through  RisingSlewLimit=SkywalkerX8.Actuators.Servos.RateLimit  FallingSlewLimit=-SkywalkerX8.Actuators.Servos.RateLimit  SampleTimeMode=inherited  InitialCondition=SkywalkerX8.InitialConditions.de*0.5 - SkywalkerX8.InitialConditions.da*0.5
  Saturation : Saturate  UpperLimit=SkywalkerX8.Actuators.Servos.UpperSaturation  LowerLimit=SkywalkerX8.Actuators.Servos.LowerSaturation
  Second Order Servo-Motor Model : simulink_extras/Additional Linear/State-Space (with initial outputs)  A=SkywalkerX8.Actuators.Servos.SS.A  B=SkywalkerX8.Actuators.Servos.SS.B  C=SkywalkerX8.Actuators.Servos.SS.C  D=SkywalkerX8.Actuators.Servos.SS.D  U0=(SkywalkerX8.InitialConditions.de*0.5 - SkywalkerX8.InitialConditions.da*0.5)  Y0=(SkywalkerX8.InitialConditions.de*0.5 - SkywalkerX8.InitialConditions.da*0.5)
      settings: SourceProductName=Simulink  SourceProductBaseCode=SL
  Terminator : Terminator
  der : Outport
  wires:
  Rate Limiter/1 -> Saturation/1
  der_c/1 -> Second Order Servo-Motor Model/1
  Second Order Servo-Motor Model/1 -> Derivative/1, Rate Limiter/1
  Saturation/1 -> der/1
  Derivative/1 -> Abs/1
  Abs/1 -> Compare To Constant/1
  Compare To Constant/1 -> Terminator/1  "rServoRateLimitCheck"

== system SkywalkerX8_Control_Observable_Feedback/Autopilot Digital/Chi Rate Limiter Dynamic ==
  note: U(k)
  note: Y(k)
  up : Inport
  u : Inport  Port=2
  lo : Inport  Port=3
  Delay Input2 : UnitDelay  Description=Store in Global RAM  DisableCoverage=on  InitialCondition=initOutput  SampleTime=-1
  Difference Inputs1 : Sum  Description=Add in CPU  DisableCoverage=on  Inputs=+-  OutDataTypeStr=Inherit: Inherit via back propagation
  Difference Inputs2 : Sum  Description=Add in CPU  OutDataTypeStr=Inherit: Inherit via back propagation
  FixPt Data Type Duplicate : DataTypeDuplicate  DisableCoverage=on  NumInputPorts=7
  Saturation Dynamic : simulink/Discontinuities/Saturation Dynamic  OutMin=[]  OutMax=[]  OutDataTypeStr=Inherit: Same as second input  OutDataType=fixdt(1, 16)  OutScaling=2^-10  DoSatur=off
  delta fall limit : Product  DisableCoverage=on  Inputs=**  OutDataTypeStr=Inherit: Inherit via back propagation  SaturateOnIntegerOverflow=on
  delta rise limit : Product  DisableCoverage=on  Inputs=**  OutDataTypeStr=Inherit: Inherit via back propagation  SaturateOnIntegerOverflow=on
  sample time : SampleTimeMath  DisableCoverage=on  TsampMathOp=Ts Only  weightValue=1
  Y : Outport  InitialOutput=0
  wires:
  Delay Input2/1 -> Difference Inputs1/2, FixPt Data Type Duplicate/2, Difference Inputs2/2  "Y(k-1)"
  Difference Inputs1/1 -> FixPt Data Type Duplicate/4, Saturation Dynamic/2  "( U(k) - Y(k-1) )"
  Difference Inputs2/1 -> Y/1, Delay Input2/1, FixPt Data Type Duplicate/1
  u/1 -> Difference Inputs1/1, FixPt Data Type Duplicate/5, sample time/1
  delta fall limit/1 -> FixPt Data Type Duplicate/3, Saturation Dynamic/3
  sample time/1 -> delta fall limit/2, delta rise limit/2
  Saturation Dynamic/1 -> Difference Inputs2/1, FixPt Data Type Duplicate/7
  delta rise limit/1 -> FixPt Data Type Duplicate/6, Saturation Dynamic/1
  lo/1 -> delta fall limit/1
  up/1 -> delta rise limit/1

== system SkywalkerX8_Control_Observable_Feedback/Autopilot Digital/Gain Scheduled Controller Chi ==
  Chi_e : Inport
  Va : Inport  Port=2
  PIDF Controller Chi Ki 2D Lookup Table : Lookup_n-D  NumberOfTableDimensions=1  BreakpointsForDimension1=SkywalkerX8.Control.Lateral.SchedulingVariables.VaArray  BreakpointsForDimension2=SkywalkerX8.Control.Longitudinal.SchedulingVariables.alphaArray  Table=SkywalkerX8.Control.Lateral.ChiController.Digital.KiChi  InternalRulePriority=Speed  RndMeth=Simplest  InputSameDT=on
  PIDF Controller Chi Kp 2D Lookup Table : Lookup_n-D  NumberOfTableDimensions=1  BreakpointsForDimension1=SkywalkerX8.Control.Lateral.SchedulingVariables.VaArray  BreakpointsForDimension2=SkywalkerX8.Control.Longitudinal.SchedulingVariables.alphaArray  Table=SkywalkerX8.Control.Lateral.ChiController.Digital.KpChi  InternalRulePriority=Speed  RndMeth=Simplest  InputSameDT=on
  PIDF Controller Va_theta : Subsystem
  Saturation : Saturate  UpperLimit=SkywalkerX8.Control.Lateral.ChiController.upperSaturationPhiC  LowerLimit=SkywalkerX8.Control.Lateral.ChiController.lowerSaturationPhiC
  Phi_c : Outport
  wires:
  PIDF Controller Chi Kp 2D Lookup Table/1 -> PIDF Controller Va_theta/2(P)
  Chi_e/1 -> PIDF Controller Va_theta/1(u)
  Va/1 -> PIDF Controller Chi Kp 2D Lookup Table/1, PIDF Controller Chi Ki 2D Lookup Table/1
  PIDF Controller Chi Ki 2D Lookup Table/1 -> PIDF Controller Va_theta/3(I)
  Saturation/1 -> PIDF Controller Va_theta/4(Post-Saturation), Phi_c/1
  PIDF Controller Va_theta/1(y) -> PIDF Controller Va_theta/5(Pre-Saturation), Saturation/1
